simulink subsystem "actuator_modelling"  (R2024a)
settings: Solver=VariableStepAuto  StartTime=0.0  StopTime=10.0  RelTol=1e-3
undefined symbols (not defined in the file or in its folder): magnotorquer_current_to_magnetic
libraries: matrix_library x1
settings Model: Creator=joshu  LastModifiedBy=joshu

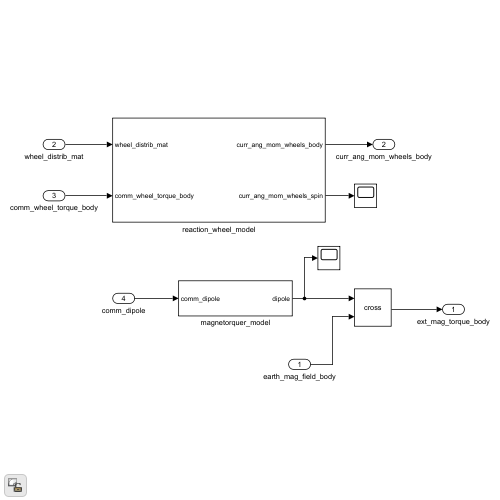
[thumbnail: Simulink's stored preview of the top-level diagram]
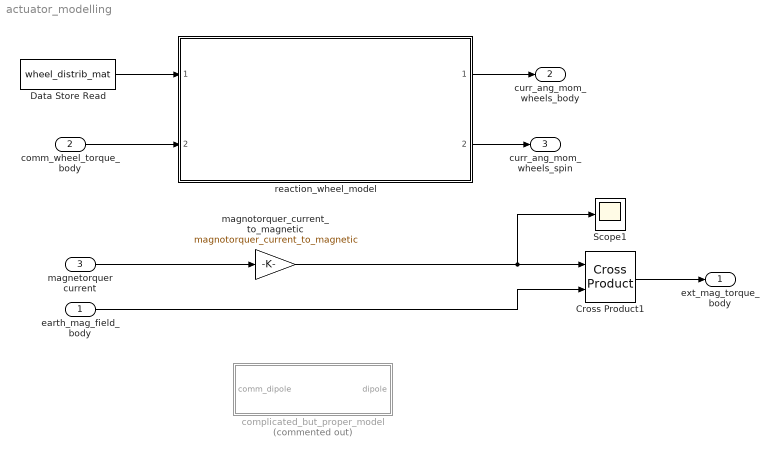
== system actuator_modelling ==
  earth_mag_field_body : Inport
  comm_wheel_torque_body : Inport  Port=2
  magnetorquer current : Inport  Port=3
  Cross Product1 : matrix_library/Cross Product
  Data Store Read : DataStoreRead  DataStoreName=wheel_distrib_mat  IndexOptions=Index vector (dialog)  Indices=1  OutputSizes=1
  Scope1 : Scope
  complicated_but_proper_model : Subsystem  Commented=on
  magnotorquer_current_to_magnetic : Gain  Gain=magnotorquer_current_to_magnetic
  reaction_wheel_model : Subsystem  ReferencedSubsystem=reaction_wheel_model
  ext_mag_torque_body : Outport
  curr_ang_mom_wheels_body : Outport  Port=2
  curr_ang_mom_wheels_spin : Outport  Port=3
  wires:
  reaction_wheel_model/2 -> curr_ang_mom_wheels_spin/1
  magnotorquer_current_to_magnetic/1 -> Cross Product1/1, Scope1/1
  Cross Product1/1 -> ext_mag_torque_body/1
  Data Store Read/1 -> reaction_wheel_model/1
  comm_wheel_torque_body/1 -> reaction_wheel_model/2
  earth_mag_field_body/1 -> Cross Product1/2
  magnetorquer current/1 -> magnotorquer_current_to_magnetic/1
  reaction_wheel_model/1 -> curr_ang_mom_wheels_body/1

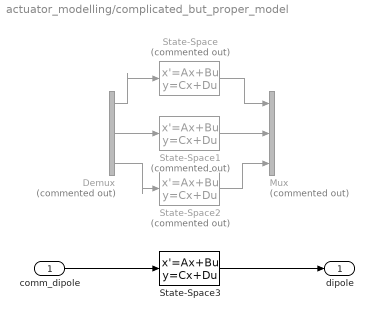
== system actuator_modelling/complicated_but_proper_model ==
  comm_dipole : Inport
  Demux : Demux  Commented=on  Outputs=3
  Mux : Mux  Commented=on  Inputs=3
  State-Space : StateSpace  Commented=on  A=-71.31  B=8  C=8.914  D=0  InitialCondition=0
  State-Space1 : StateSpace  Commented=on  A=-71.31  B=8  C=8.914  D=0  InitialCondition=0
  State-Space2 : StateSpace  Commented=on  A=-71.31  B=8  C=8.914  D=0  InitialCondition=0
  State-Space3 : StateSpace  A=eye(3)*-71.31  B=eye(3)*8  C=eye(3)*8.914  D=zeros(3)  InitialCondition=[0 0 0]
  dipole : Outport
  wires:
  comm_dipole/1 -> State-Space3/1
  State-Space3/1 -> dipole/1
  Demux/3 -> State-Space2/1
  Demux/1 -> State-Space/1
  Demux/2 -> State-Space1/1
  State-Space1/1 -> Mux/2
  State-Space2/1 -> Mux/3
  State-Space/1 -> Mux/1
